simulink model "Model"  (R2020b)
settings: Solver=FixedStepDiscrete  StartTime=0.0  StopTime=50.0  FixedStep=1  RelTol=1e-3
libraries: dspvision x2, dspsnks4 x1
settings Model: Creator=Nic  LastModifiedBy=Nic

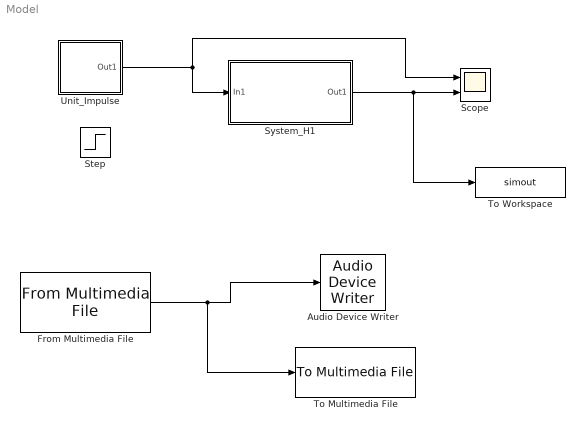
== system Model ==
  Audio Device Writer : dspsnks4/Audio Device Writer  Driver=DirectSound  Device=Default  InheritSampleRate=on  SampleRate=44100  BitDepth=16-bit integer  BufferSize=4096  NumBuffers=10  DefaultOutputChannelMapping=on  OutputChannelMapping=1:2  OutputNumUnderrunSamples=off  DriverIdx=1  DeviceWarnFlag=''
  From Multimedia File : dspvision/From Multimedia File  inputFilename=speech_dft.mp3  readRange=[1 Inf]  loop=on  numPlays=inf  outputStreams=Audio only  videoDataType=single  audioDataType=double  inheritSampleTime=on  userDefinedSampleTime=1/30  noAudioOutput=off  isIntensityVideo=off  fourcc=RGB  colorVideoFormat=Separate color signals  outputEOF=off  dataOrg=Column-major  audioFrameSize=1024  computeAudioFrameSize=off  outSamplingMode=Sample based
  Scope : Scope  NumInputPorts=2
  Step : Step  SampleTime=0
  System_H1 : Subsystem
  To Multimedia File : dspvision/To Multimedia File  outputFilename=output.wav  streamSelection=Audio only  videoCompressor=None (uncompressed)  audioCompressor=None (uncompressed)  imagePorts=Separate color signals  fileType=WAV  audioDatatype=16-bit integer  fourcc=RGB  videoQuality=75  mj2000CompFactor=10
  To Workspace : ToWorkspace  VariableName=simout  SampleTime=-1
  Unit_Impulse : Subsystem
  wires:
  System_H1/1(Out1) -> To Workspace/1, Scope/2
  Unit_Impulse/1(Out1) -> System_H1/1(In1), Scope/1
  From Multimedia File/1 -> To Multimedia File/1, Audio Device Writer/1

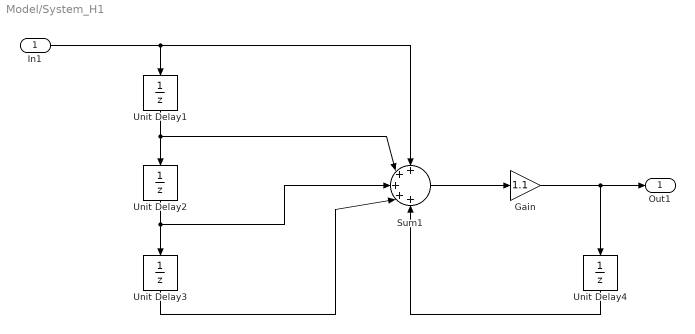
== system Model/System_H1 ==
  In1 : Inport
  Gain : Gain  Gain=1.1
  Sum1 : Sum  Inputs=+++++
  Unit Delay{1..4} (4 alike) : UnitDelay  SampleTime=-1  HasFrameUpgradeWarning=on
  Out1 : Outport
  wires:
  Sum1/1 -> Gain/1
  In1/1 -> Sum1/1, Unit Delay1/1
  Unit Delay1/1 -> Unit Delay2/1, Sum1/2
  Unit Delay3/1 -> Sum1/4
  Unit Delay2/1 -> Unit Delay3/1, Sum1/3
  Gain/1 -> Unit Delay4/1, Out1/1
  Unit Delay4/1 -> Sum1/5

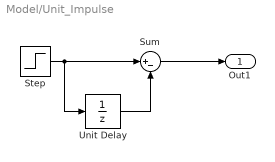
== system Model/Unit_Impulse ==
  Step : Step  SampleTime=0
  Sum : Sum  Inputs=|+-
  Unit Delay : UnitDelay  SampleTime=-1  HasFrameUpgradeWarning=on
  Out1 : Outport
  wires:
  Unit Delay/1 -> Sum/2
  Sum/1 -> Out1/1
  Step/1 -> Unit Delay/1, Sum/1
